simulink model "robust_tracking_nicolas"  (R2020b)
settings: Solver=VariableStepAuto  StartTime=0.0  StopTime=40.0  RelTol=1e-3
values from neighbouring files (symbols this model uses):
  drv =     [balrob_params.mat]
  g = 9.81    [balrob_params.mat]    (also in sfun_balrob_long_dyn.m)
  gbox =     [balrob_params.mat]    (also in sfun_balrob_long_dyn.m = block.DialogPrm(4).Data)
  ms22g = 0.101936799185    [balrob_params.mat]
  sens =     [balrob_params.mat]
  Ts = 0.01    [balrob_params.mat]
  wheel =     [balrob_params.mat]    (also in sfun_balrob_long_dyn.m = block.DialogPrm(5).Data)
undefined symbols (not defined in the file or in its folder): C12qq_coeff, C_gain, denHw, denLPFz, DiscIntNeverNeededParam, Fv1, g2_coeff, Ki, M11q, M12q_coeff, M22q, N_u, N_x, numHw, numLPFz, step_disturbance, step_size, T, ua2tau1
settings Model: Creator=39345  LastModifiedBy=39345
settings DataIOCC: ReturnWorkspaceOutputs=off

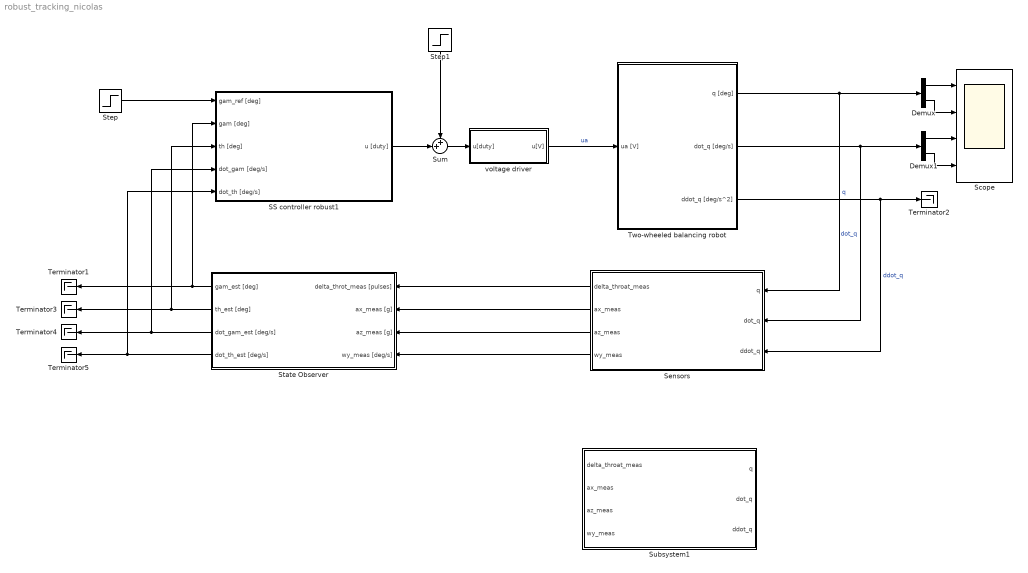
== system robust_tracking_nicolas ==
  Demux : Demux  Outputs=2
  Demux1 : Demux  Outputs=2
  SS controller robust1 : Subsystem
  Scope : Scope  NumInputPorts=4
  Sensors : Subsystem
  State Observer : Subsystem
  Step : Step  After=step_size  SampleTime=0.01
  Step1 : Step  Time=11  After=step_disturbance  SampleTime=0.01
  Subsystem1 : Subsystem
  Sum : Sum  Inputs=++|
  Terminator{1..5} (5 alike) : Terminator
  Two-wheeled balancing robot : Subsystem
  voltage driver : Subsystem
  wires:
  SS controller robust1/1(u [duty]) -> Sum/2
  State Observer/1(gam_est [deg]) -> SS controller robust1/2(gam [deg]), Terminator1/1
  State Observer/2(th_est [deg]) -> SS controller robust1/3(th [deg]), Terminator3/1
  State Observer/3(dot_gam_est [deg/s]) -> SS controller robust1/4(dot_gam [deg/s]), Terminator4/1
  State Observer/4(dot_th_est [deg/s]) -> SS controller robust1/5(dot_th [deg/s]), Terminator5/1
  Sum/1 -> voltage driver/1(u[duty])
  Demux1/1 -> Scope/3
  Sensors/1(delta_throat_meas) -> State Observer/1("delta_throt_meas [pulses] ")
  Sensors/4(wy_meas) -> State Observer/4(wy_meas [deg/s])
  Two-wheeled balancing robot/3(ddot_q [deg/s^2]) -> Sensors/3(ddot_q), Terminator2/1  "ddot_q"
  voltage driver/1(u[V]) -> Two-wheeled balancing robot/1(ua [V])  "ua"
  Demux/2 -> Scope/2
  Sensors/3(az_meas) -> State Observer/3("az_meas [g] ")
  Two-wheeled balancing robot/2(dot_q [deg/s]) -> Sensors/2(dot_q), Demux1/1  "dot_q"
  Demux1/2 -> Scope/4
  Demux/1 -> Scope/1
  Sensors/2(ax_meas) -> State Observer/2("ax_meas [g] ")
  Two-wheeled balancing robot/1(q [deg]) -> Sensors/1(q), Demux/1  "q"
  Step/1 -> SS controller robust1/1(gam_ref [deg])
  Step1/1 -> Sum/1

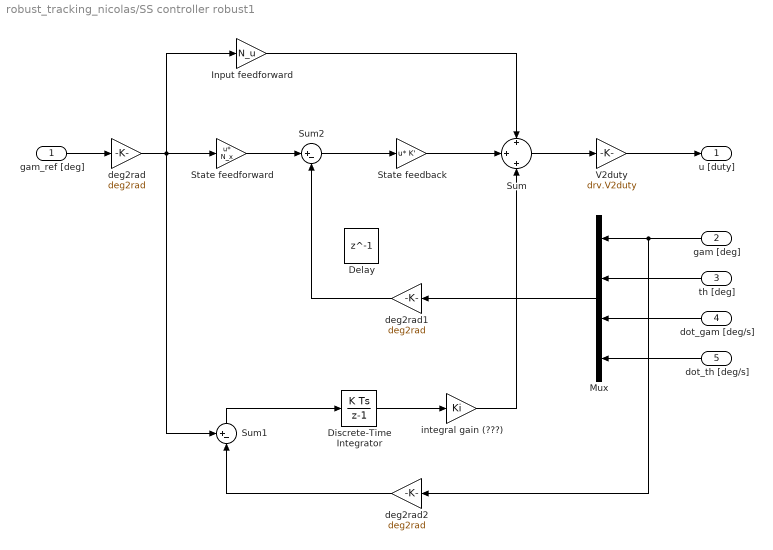
== system robust_tracking_nicolas/SS controller robust1 ==
  gam_ref [deg] : Inport
  gam [deg] : Inport  Port=2
  th [deg] : Inport  Port=3
  dot_gam [deg/s] : Inport  Port=4
  dot_th [deg/s] : Inport  Port=5
  Delay : Delay  DelayLength=1  InitialCondition=0
  Discrete-Time Integrator : DiscreteIntegrator  SampleTime=-1  ICPrevOutput=DiscIntNeverNeededParam  ICPrevScaledInput=DiscIntNeverNeededParam
  Input feedforward : Gain  Gain=N_u
  Mux : Mux
  State feedback : Gain  Gain=K'  Multiplication=Matrix(u*K)
  "State feedforward\t" : Gain  Gain=N_x  Multiplication=Matrix(u*K)
  Sum : Sum  Inputs=+|+|+
  Sum1 : Sum  Inputs=+-|
  Sum2 : Sum  Inputs=|+-
  V2duty : Gain  Gain=drv.V2duty
  deg2rad : Gain  Gain=deg2rad
  deg2rad1 : Gain  Gain=deg2rad
  deg2rad2 : Gain  Gain=deg2rad
  integral gain (???) : Gain  Gain=Ki
  u [duty] : Outport
  wires:
  gam_ref [deg]/1 -> deg2rad/1
  deg2rad/1 -> Sum1/1, "State feedforward\t"/1, Input feedforward/1
  State feedback/1 -> Sum/2
  "State feedforward\t"/1 -> Sum2/1
  Sum2/1 -> State feedback/1
  Input feedforward/1 -> Sum/1
  Sum/1 -> V2duty/1
  V2duty/1 -> u [duty]/1
  gam [deg]/1 -> deg2rad2/1, Mux/1
  Mux/1 -> deg2rad1/1
  dot_gam [deg/s]/1 -> Mux/3
  th [deg]/1 -> Mux/2
  dot_th [deg/s]/1 -> Mux/4
  deg2rad1/1 -> Sum2/2
  deg2rad2/1 -> Sum1/2
  Sum1/1 -> Discrete-Time Integrator/1
  Discrete-Time Integrator/1 -> integral gain (???)/1
  integral gain (???)/1 -> Sum/3

== system robust_tracking_nicolas/Sensors ==
  q : Inport
  dot_q : Inport  Port=2
  ddot_q : Inport  Port=3
  MPU : Subsystem
  encoder : Subsystem
  delta_throat_meas : Outport
  ax_meas : Outport  Port=2
  az_meas : Outport  Port=3
  wy_meas : Outport  Port=4
  wires:
  MPU/2(az[g]) -> az_meas/1  "az_meas"
  MPU/3(wy[deg/s]) -> wy_meas/1  "wy_meas"
  q/1 -> MPU/1(q [deg]), encoder/1(q[deg])
  ddot_q/1 -> MPU/3(ddot_q[deg/s^2])
  encoder/1(delta_throt[pulses]) -> delta_throat_meas/1  "delta_throat_meas"
  dot_q/1 -> MPU/2(dot_q [deg/s])
  MPU/1(ax[g]) -> ax_meas/1  "ax_meas"

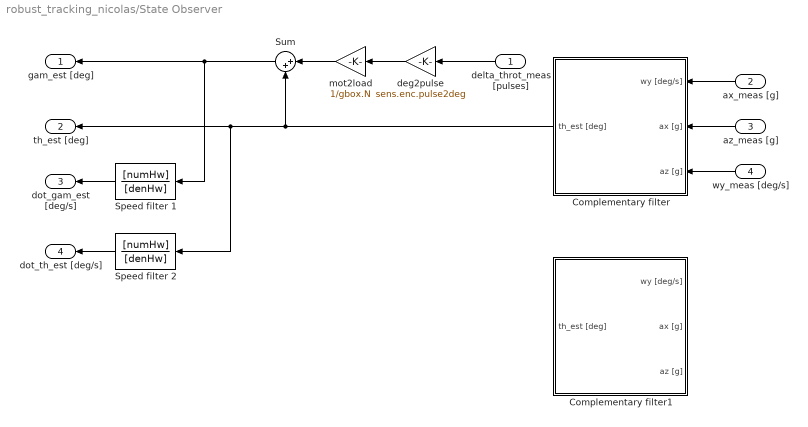
== system robust_tracking_nicolas/State Observer ==
  "delta_throt_meas [pulses] " : Inport
  "ax_meas [g] " : Inport  Port=2
  "az_meas [g] " : Inport  Port=3
  wy_meas [deg/s] : Inport  Port=4
  Complementary filter : Subsystem
  Complementary filter1 : Subsystem
  Speed filter 1 : DiscreteTransferFcn  Numerator=[numHw]  Denominator=[denHw]
  Speed filter 2 : DiscreteTransferFcn  Numerator=[numHw]  Denominator=[denHw]
  Sum : Sum  Inputs=|++
  deg2pulse : Gain  Gain=sens.enc.pulse2deg
  mot2load : Gain  Gain=1/gbox.N
  gam_est [deg] : Outport
  th_est [deg] : Outport  Port=2
  dot_gam_est [deg/s] : Outport  Port=3
  dot_th_est [deg/s] : Outport  Port=4
  wires:
  "ax_meas [g] "/1 -> Complementary filter/1(wy [deg/s])
  "az_meas [g] "/1 -> Complementary filter/2("ax [g] ")
  wy_meas [deg/s]/1 -> Complementary filter/3("az [g] ")
  deg2pulse/1 -> mot2load/1
  "delta_throt_meas [pulses] "/1 -> deg2pulse/1
  mot2load/1 -> Sum/1
  Complementary filter/1("th_est [deg] ") -> Sum/2, Speed filter 2/1, th_est [deg]/1
  Sum/1 -> Speed filter 1/1, gam_est [deg]/1
  Speed filter 1/1 -> dot_gam_est [deg/s]/1
  Speed filter 2/1 -> dot_th_est [deg/s]/1

== system robust_tracking_nicolas/Subsystem1 ==
  q : Inport
  dot_q : Inport  Port=2
  ddot_q : Inport  Port=3
  MPU : Subsystem
  encoder : Subsystem
  delta_throat_meas : Outport
  ax_meas : Outport  Port=2
  az_meas : Outport  Port=3
  wy_meas : Outport  Port=4
  wires:
  MPU/2(az[g]) -> az_meas/1  "az_meas"
  MPU/3(wy[deg/s]) -> wy_meas/1  "wy_meas"
  q/1 -> MPU/1(q [deg]), encoder/1(q[deg])
  ddot_q/1 -> MPU/3(ddot_q[deg/s^2])
  encoder/1(delta_throt[pulses]) -> delta_throat_meas/1  "delta_throat_meas"
  dot_q/1 -> MPU/2(dot_q [deg/s])
  MPU/1(ax[g]) -> ax_meas/1  "ax_meas"

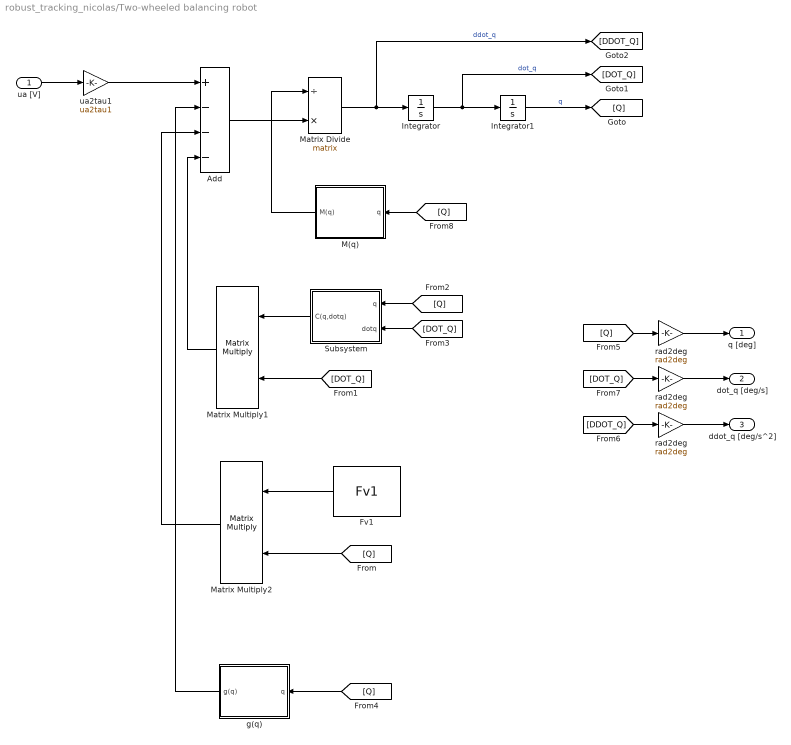
== system robust_tracking_nicolas/Two-wheeled balancing robot ==
  ua [V] : Inport
  Add : Sum  Inputs=+---
  Fv1 : Constant  Value=Fv1
  Integrator : Integrator
  Integrator1 : Integrator
  M(q) : Subsystem
  Matrix Divide : Product  Inputs=/*  Multiplication=Matrix(*)
  Matrix Multiply1 : Product  Multiplication=Matrix(*)
  Matrix Multiply2 : Product  Multiplication=Matrix(*)
  Subsystem : Subsystem
  g(q) : Subsystem
  rad2deg : Gain  Gain=rad2deg
  "rad2deg " : Gain  Gain=rad2deg
  "rad2deg  " : Gain  Gain=rad2deg
  ua2tau1 : Gain  Gain=ua2tau1
  q [deg] : Outport
  dot_q [deg/s] : Outport  Port=2
  ddot_q [deg/s^2] : Outport  Port=3
  wires:
  [DOT_Q] -> "rad2deg  "/1
  [DDOT_Q] -> "rad2deg "/1
  [Q] -> rad2deg/1
  "rad2deg  "/1 -> dot_q [deg/s]/1
  rad2deg/1 -> q [deg]/1
  "rad2deg "/1 -> ddot_q [deg/s^2]/1
  Matrix Divide/1 -> [DDOT_Q], Integrator/1  "ddot_q"
  Add/1 -> Matrix Divide/2
  [Q] -> M(q)/1(q)
  Integrator1/1 -> [Q]  "q"
  [Q] -> Subsystem/1(q)
  ua2tau1/1 -> Add/1
  Subsystem/1(C(q,dotq)) -> Matrix Multiply1/1
  [Q] -> g(q)/1(q)
  Matrix Multiply1/1 -> Add/4
  Integrator/1 -> [DOT_Q], Integrator1/1  "dot_q"
  g(q)/1(g(q)) -> Add/2
  [Q] -> Matrix Multiply2/2
  Matrix Multiply2/1 -> Add/3
  M(q)/1(M(q)) -> Matrix Divide/1
  [DOT_Q] -> Matrix Multiply1/2
  Fv1/1 -> Matrix Multiply2/1
  [DOT_Q] -> Subsystem/2(dotq)
  ua [V]/1 -> ua2tau1/1

== system robust_tracking_nicolas/voltage driver ==
  u[duty] : Inport
  Rounding Function : Rounding  Operator=fix
  Zero-Order Hold : ZeroOrderHold  SampleTime=Ts
  duty saturation : Saturate  UpperLimit=drv.dutymax  LowerLimit=-drv.dutymax
  duty2V : Gain  Gain=drv.duty2V
  voltage saturation1 : Saturate  UpperLimit=drv.Vbus  LowerLimit=-drv.Vbus
  u[V] : Outport
  wires:
  u[duty]/1 -> duty saturation/1
  duty saturation/1 -> Rounding Function/1
  Rounding Function/1 -> duty2V/1
  duty2V/1 -> voltage saturation1/1
  voltage saturation1/1 -> Zero-Order Hold/1
  Zero-Order Hold/1 -> u[V]/1

== system robust_tracking_nicolas/Sensors/MPU ==
  q [deg] : Inport
  dot_q [deg/s] : Inport  Port=2
  ddot_q[deg/s^2] : Inport  Port=3
  Accelerometer : Subsystem
  Gyroscope : Subsystem
  ax[g] : Outport
  az[g] : Outport  Port=2
  wy[deg/s] : Outport  Port=3
  wires:
  q [deg]/1 -> Accelerometer/1(q [deg])
  dot_q [deg/s]/1 -> Gyroscope/1(dot_q [deg/s]), Accelerometer/2(dot_q [deg/s])
  ddot_q[deg/s^2]/1 -> Accelerometer/3(ddot_q[deg/s^2])
  Gyroscope/1(wy[deg/s]) -> wy[deg/s]/1
  Accelerometer/1(ax[g]) -> ax[g]/1
  Accelerometer/2(az[g]) -> az[g]/1

== system robust_tracking_nicolas/Sensors/encoder ==
  q[deg] : Inport
  Demux : Demux  Outputs=2
  Subtract : Sum  Inputs=+-
  deg2pulse : Gain  Gain=sens.enc.deg2pulse
  encoder quantization : Quantizer  QuantizationInterval=sens.enc.pulse2deg
  encoder sampling : ZeroOrderHold  SampleTime=Ts
  load2mot : Gain  Gain=gbox.N
  delta_throt[pulses] : Outport
  wires:
  q[deg]/1 -> Demux/1
  Demux/1 -> Subtract/1  "gam"
  Demux/2 -> Subtract/2  "th"
  Subtract/1 -> load2mot/1
  load2mot/1 -> encoder sampling/1  "delta_throt"
  encoder sampling/1 -> encoder quantization/1
  encoder quantization/1 -> deg2pulse/1
  deg2pulse/1 -> delta_throt[pulses]/1

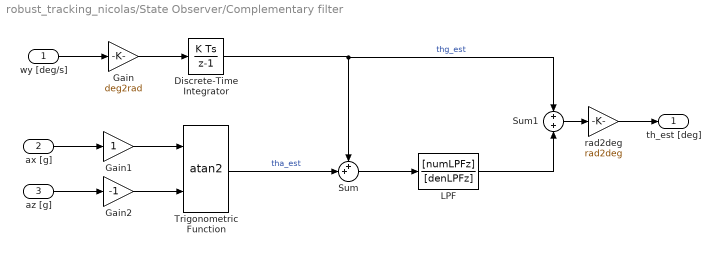
== system robust_tracking_nicolas/State Observer/Complementary filter ==
  wy [deg/s] : Inport
  "ax [g] " : Inport  Port=2
  "az [g] " : Inport  Port=3
  Discrete-Time Integrator : DiscreteIntegrator  gainval=1  SampleTime=Ts  ICPrevOutput=DiscIntNeverNeededParam  ICPrevScaledInput=DiscIntNeverNeededParam
  Gain : Gain  Gain=deg2rad
  Gain1 : Gain
  Gain2 : Gain  Gain=-1
  LPF : DiscreteTransferFcn  Numerator=[numLPFz]  Denominator=[denLPFz]
  Sum : Sum  Inputs=++|
  Sum1 : Sum
  Trigonometric Function : Trigonometry  Operator=atan2
  rad2deg : Gain  Gain=rad2deg
  "th_est [deg] " : Outport
  wires:
  "az [g] "/1 -> Gain2/1
  "ax [g] "/1 -> Gain1/1
  wy [deg/s]/1 -> Gain/1
  Gain/1 -> Discrete-Time Integrator/1
  Gain2/1 -> Trigonometric Function/2
  Gain1/1 -> Trigonometric Function/1
  Trigonometric Function/1 -> Sum/2  "tha_est"
  Discrete-Time Integrator/1 -> Sum1/1, Sum/1  "thg_est"
  rad2deg/1 -> "th_est [deg] "/1
  Sum1/1 -> rad2deg/1
  Sum/1 -> LPF/1
  LPF/1 -> Sum1/2

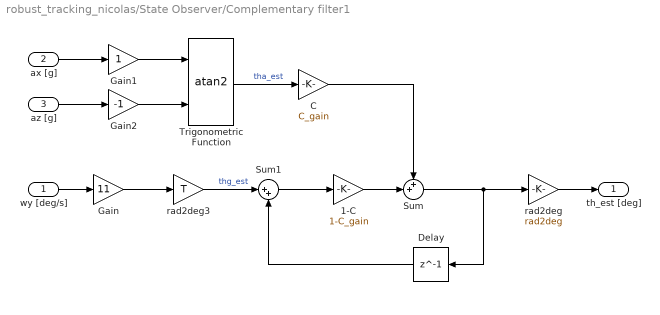
== system robust_tracking_nicolas/State Observer/Complementary filter1 ==
  wy [deg/s] : Inport
  "ax [g] " : Inport  Port=2
  "az [g] " : Inport  Port=3
  1-C : Gain  Gain=1-C_gain
  C : Gain  Gain=C_gain
  Delay : Delay  DelayLength=1
  Gain : Gain  Gain=11
  Gain1 : Gain
  Gain2 : Gain  Gain=-1
  Sum : Sum  Inputs=++|
  Sum1 : Sum  Inputs=|++
  Trigonometric Function : Trigonometry  Operator=atan2
  rad2deg : Gain  Gain=rad2deg
  rad2deg3 : Gain  Gain=T
  "th_est [deg] " : Outport
  wires:
  "az [g] "/1 -> Gain2/1
  "ax [g] "/1 -> Gain1/1
  wy [deg/s]/1 -> Gain/1
  Gain/1 -> rad2deg3/1
  Gain2/1 -> Trigonometric Function/2
  Gain1/1 -> Trigonometric Function/1
  rad2deg/1 -> "th_est [deg] "/1
  Trigonometric Function/1 -> C/1  "tha_est"
  C/1 -> Sum/1
  1-C/1 -> Sum/2
  Sum/1 -> Delay/1, rad2deg/1
  Delay/1 -> Sum1/2
  rad2deg3/1 -> Sum1/1  "thg_est"
  Sum1/1 -> 1-C/1

== system robust_tracking_nicolas/Subsystem1/MPU ==
  q [deg] : Inport
  dot_q [deg/s] : Inport  Port=2
  ddot_q[deg/s^2] : Inport  Port=3
  Accelerometer : Subsystem
  Gyroscope : Subsystem
  ax[g] : Outport
  az[g] : Outport  Port=2
  wy[deg/s] : Outport  Port=3
  wires:
  q [deg]/1 -> Accelerometer/1(q [deg])
  dot_q [deg/s]/1 -> Gyroscope/1(dot_q [deg/s]), Accelerometer/2(dot_q [deg/s])
  ddot_q[deg/s^2]/1 -> Accelerometer/3(ddot_q[deg/s^2])
  Gyroscope/1(wy[deg/s]) -> wy[deg/s]/1
  Accelerometer/1(ax[g]) -> ax[g]/1
  Accelerometer/2(az[g]) -> az[g]/1

== system robust_tracking_nicolas/Subsystem1/encoder ==
  q[deg] : Inport
  Demux : Demux  Outputs=2
  Subtract : Sum  Inputs=+-
  deg2pulse : Gain  Gain=sens.enc.deg2pulse
  encoder quantization : Quantizer  QuantizationInterval=sens.enc.pulse2deg
  encoder sampling : ZeroOrderHold  SampleTime=Ts
  load2mot : Gain  Gain=gbox.N
  delta_throt[pulses] : Outport
  wires:
  q[deg]/1 -> Demux/1
  Demux/1 -> Subtract/1  "gam"
  Demux/2 -> Subtract/2  "th"
  Subtract/1 -> load2mot/1
  load2mot/1 -> encoder sampling/1  "delta_throt"
  encoder sampling/1 -> encoder quantization/1
  encoder quantization/1 -> deg2pulse/1
  deg2pulse/1 -> delta_throt[pulses]/1

== system robust_tracking_nicolas/Two-wheeled balancing robot/M(q) ==
  q : Inport
  Constant : Constant  Value=M11q
  Constant1 : Constant  Value=M22q
  Function Caller : FunctionCaller  FunctionPrototype=y = M12q(u)  InputArgumentSpecifications=<Enter example>  OutputArgumentSpecifications=<Enter example>
  Matrix Concatenate1 : Concatenate  Mode=Multidimensional array  ConcatenateDimension=2
  Mux : Mux  Inputs=2
  Mux1 : Mux  Inputs=2
  Selector1 : Selector  InputPortWidth=2  IndexOptions=Index vector (dialog)  Indices=2  OutputSizes=1
  Simulink Function : Subsystem  TreatAsAtomicUnit=on
  M(q) : Outport
  wires:
  q/1 -> Selector1/1
  Mux1/1 -> Matrix Concatenate1/2
  Constant1/1 -> Mux1/2
  Mux/1 -> Matrix Concatenate1/1
  Function Caller/1 -> Mux/2, Mux1/1
  Matrix Concatenate1/1 -> M(q)/1
  Selector1/1 -> Function Caller/1
  Constant/1 -> Mux/1

== system robust_tracking_nicolas/Two-wheeled balancing robot/Subsystem ==
  q : Inport
  dotq : Inport  Port=2
  Constant : Constant  Value=0
  Gain : Gain  Gain=C12qq_coeff
  Matrix Concatenate1 : Concatenate  Mode=Multidimensional array  ConcatenateDimension=2
  Mux2 : Mux  Inputs=2
  Mux3 : Mux  Inputs=2
  Product : Product
  Selector1 : Selector  InputPortWidth=2  IndexOptions=Index vector (dialog)  Indices=2  OutputSizes=1
  Selector2 : Selector  InputPortWidth=2  IndexOptions=Index vector (dialog)  Indices=2  OutputSizes=1
  Trigonometric Function : Trigonometry
  C(q,dotq) : Outport
  wires:
  Mux3/1 -> Matrix Concatenate1/2
  Mux2/1 -> Matrix Concatenate1/1
  Constant/1 -> Mux3/2, Mux2/2, Mux2/1
  Matrix Concatenate1/1 -> C(q,dotq)/1
  Gain/1 -> Mux3/1
  q/1 -> Selector2/1
  dotq/1 -> Selector1/1
  Selector1/1 -> Product/2
  Product/1 -> Gain/1
  Trigonometric Function/1 -> Product/1
  Selector2/1 -> Trigonometric Function/1

== system robust_tracking_nicolas/Two-wheeled balancing robot/g(q) ==
  q : Inport
  Constant : Constant  Value=0
  Function Caller : FunctionCaller  FunctionPrototype=y = g2(u)  InputArgumentSpecifications=<Enter example>  OutputArgumentSpecifications=<Enter example>
  Mux : Mux  Inputs=2
  Selector1 : Selector  InputPortWidth=2  IndexOptions=Index vector (dialog)  Indices=2  OutputSizes=1
  Simulink Function : Subsystem  TreatAsAtomicUnit=on
  g(q) : Outport
  wires:
  q/1 -> Selector1/1
  Selector1/1 -> Function Caller/1
  Constant/1 -> Mux/1
  Function Caller/1 -> Mux/2
  Mux/1 -> g(q)/1

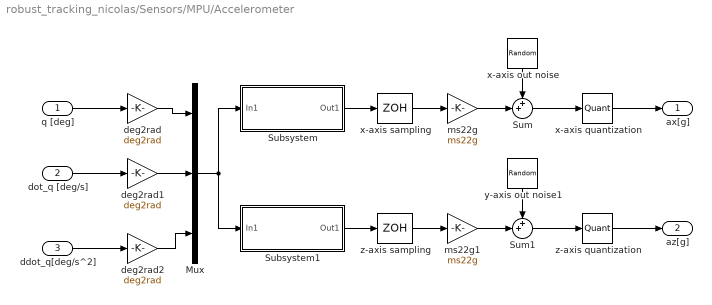
== system robust_tracking_nicolas/Sensors/MPU/Accelerometer ==
  q [deg] : Inport
  dot_q [deg/s] : Inport  Port=2
  ddot_q[deg/s^2] : Inport  Port=3
  Mux : Mux  Inputs=3
  Subsystem : Subsystem
  Subsystem1 : Subsystem
  Sum : Sum  Inputs=++|
  Sum1 : Sum  Inputs=++|
  deg2rad : Gain  Gain=deg2rad
  deg2rad1 : Gain  Gain=deg2rad
  deg2rad2 : Gain  Gain=deg2rad
  ms22g : Gain  Gain=ms22g
  ms22g1 : Gain  Gain=ms22g
  x-axis out noise : RandomNumber  Variance=sens.mpu.acc.noisevar  SampleTime=Ts
  x-axis quantization : Quantizer  QuantizationInterval=sens.mpu.acc.LSB2g
  x-axis sampling : ZeroOrderHold  SampleTime=Ts
  y-axis out noise1 : RandomNumber  Variance=sens.mpu.acc.noisevar  SampleTime=Ts
  z-axis quantization : Quantizer  QuantizationInterval=sens.mpu.acc.LSB2g
  z-axis sampling : ZeroOrderHold  SampleTime=Ts
  ax[g] : Outport
  az[g] : Outport  Port=2
  wires:
  ddot_q[deg/s^2]/1 -> deg2rad2/1
  dot_q [deg/s]/1 -> deg2rad1/1
  q [deg]/1 -> deg2rad/1
  deg2rad2/1 -> Mux/3
  deg2rad1/1 -> Mux/2
  deg2rad/1 -> Mux/1
  x-axis sampling/1 -> ms22g/1
  z-axis sampling/1 -> ms22g1/1
  x-axis out noise/1 -> Sum/1
  ms22g/1 -> Sum/2
  y-axis out noise1/1 -> Sum1/1
  ms22g1/1 -> Sum1/2
  Sum/1 -> x-axis quantization/1
  Sum1/1 -> z-axis quantization/1
  z-axis quantization/1 -> az[g]/1
  x-axis quantization/1 -> ax[g]/1
  Mux/1 -> Subsystem1/1(In1), Subsystem/1(In1)
  Subsystem/1(Out1) -> x-axis sampling/1
  Subsystem1/1(Out1) -> z-axis sampling/1

== system robust_tracking_nicolas/Sensors/MPU/Gyroscope ==
  dot_q [deg/s] : Inport
  Random Number : RandomNumber  Variance=sens.mpu.gyro.noisevar  SampleTime=Ts
  Selector2 : Selector  InputPortWidth=2  IndexOptions=Index vector (dialog)  Indices=2  OutputSizes=1
  Sum : Sum  Inputs=++|
  y-axis quantization : Quantizer  QuantizationInterval=sens.mpu.gyro.LSB2degs
  y-axis sampling : ZeroOrderHold  SampleTime=Ts
  wy[deg/s] : Outport
  wires:
  dot_q [deg/s]/1 -> Selector2/1
  Selector2/1 -> y-axis sampling/1
  y-axis sampling/1 -> Sum/2
  Random Number/1 -> Sum/1
  Sum/1 -> y-axis quantization/1
  y-axis quantization/1 -> wy[deg/s]/1

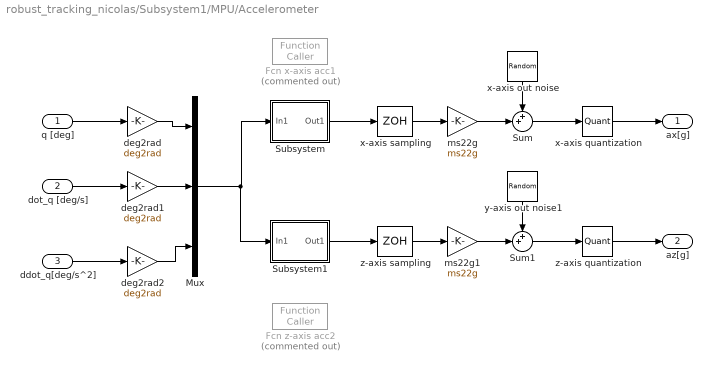
== system robust_tracking_nicolas/Subsystem1/MPU/Accelerometer ==
  q [deg] : Inport
  dot_q [deg/s] : Inport  Port=2
  ddot_q[deg/s^2] : Inport  Port=3
  Fcn x-axis acc1 : FunctionCaller  Commented=on  FunctionPrototype=y = f(u)  InputArgumentSpecifications=<Enter example>  OutputArgumentSpecifications=<Enter example>
  Fcn z-axis acc2 : FunctionCaller  Commented=on  FunctionPrototype=y = f(u)  InputArgumentSpecifications=<Enter example>  OutputArgumentSpecifications=<Enter example>
  Mux : Mux  Inputs=3
  Subsystem : Subsystem
  Subsystem1 : Subsystem
  Sum : Sum  Inputs=++|
  Sum1 : Sum  Inputs=++|
  deg2rad : Gain  Gain=deg2rad
  deg2rad1 : Gain  Gain=deg2rad
  deg2rad2 : Gain  Gain=deg2rad
  ms22g : Gain  Gain=ms22g
  ms22g1 : Gain  Gain=ms22g
  x-axis out noise : RandomNumber  Variance=sens.mpu.acc.noisevar  SampleTime=Ts
  x-axis quantization : Quantizer  QuantizationInterval=sens.mpu.acc.LSB2g
  x-axis sampling : ZeroOrderHold  SampleTime=Ts
  y-axis out noise1 : RandomNumber  Variance=sens.mpu.acc.noisevar  SampleTime=Ts
  z-axis quantization : Quantizer  QuantizationInterval=sens.mpu.acc.LSB2g
  z-axis sampling : ZeroOrderHold  SampleTime=Ts
  ax[g] : Outport
  az[g] : Outport  Port=2
  wires:
  ddot_q[deg/s^2]/1 -> deg2rad2/1
  dot_q [deg/s]/1 -> deg2rad1/1
  q [deg]/1 -> deg2rad/1
  deg2rad2/1 -> Mux/3
  deg2rad1/1 -> Mux/2
  deg2rad/1 -> Mux/1
  Mux/1 -> Subsystem1/1(In1), Subsystem/1(In1)
  Subsystem1/1(Out1) -> z-axis sampling/1
  Subsystem/1(Out1) -> x-axis sampling/1
  x-axis sampling/1 -> ms22g/1
  z-axis sampling/1 -> ms22g1/1
  x-axis out noise/1 -> Sum/1
  ms22g/1 -> Sum/2
  y-axis out noise1/1 -> Sum1/1
  ms22g1/1 -> Sum1/2
  Sum/1 -> x-axis quantization/1
  Sum1/1 -> z-axis quantization/1
  z-axis quantization/1 -> az[g]/1
  x-axis quantization/1 -> ax[g]/1

== system robust_tracking_nicolas/Subsystem1/MPU/Gyroscope ==
  dot_q [deg/s] : Inport
  Random Number : RandomNumber  Variance=sens.mpu.gyro.noisevar  SampleTime=Ts
  Selector1 : Selector  InputPortWidth=3  IndexOptions=Index vector (dialog)  Indices=[1 3]  OutputSizes=1
  Sum : Sum  Inputs=++|
  y-axis quantization : Quantizer  QuantizationInterval=sens.mpu.gyro.LSB2degs
  y-axis sampling : ZeroOrderHold  SampleTime=Ts
  wy[deg/s] : Outport
  wires:
  dot_q [deg/s]/1 -> Selector1/1
  Selector1/1 -> y-axis sampling/1
  y-axis sampling/1 -> Sum/2
  Random Number/1 -> Sum/1
  Sum/1 -> y-axis quantization/1
  y-axis quantization/1 -> wy[deg/s]/1

== system robust_tracking_nicolas/Two-wheeled balancing robot/M(q)/Simulink Function ==
  f : TriggerPort  TriggerType=function-call  IsSimulinkFunction=on  FunctionName=M12q  FunctionVisibility=scoped  VariantControl=(inherit)
  Gain : Gain  Gain=M12q_coeff
  Trigonometric Function : Trigonometry  Operator=cos
  u : ArgIn  DisableCoverage=on  ArgumentName=u
  y : ArgOut  DisableCoverage=on  ArgumentName=y
  wires:
  u/1 -> Trigonometric Function/1
  Trigonometric Function/1 -> Gain/1
  Gain/1 -> y/1

== system robust_tracking_nicolas/Two-wheeled balancing robot/g(q)/Simulink Function ==
  f : TriggerPort  TriggerType=function-call  IsSimulinkFunction=on  FunctionName=g2  FunctionVisibility=scoped  VariantControl=(inherit)
  Gain : Gain  Gain=g2_coeff
  Trigonometric Function : Trigonometry
  u : ArgIn  DisableCoverage=on  ArgumentName=u
  y : ArgOut  DisableCoverage=on  ArgumentName=y
  wires:
  u/1 -> Trigonometric Function/1
  Trigonometric Function/1 -> Gain/1
  Gain/1 -> y/1

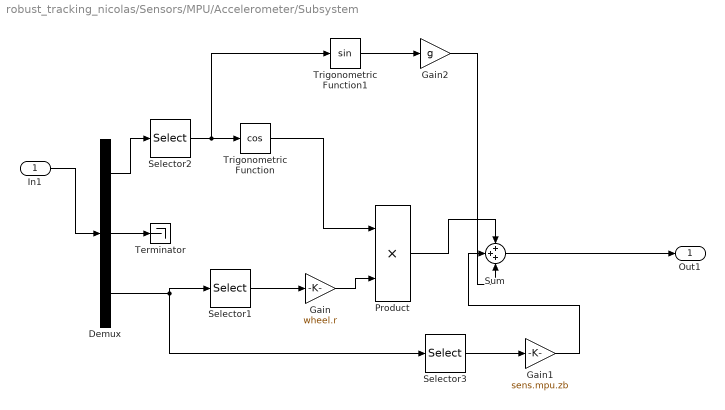
== system robust_tracking_nicolas/Sensors/MPU/Accelerometer/Subsystem ==
  In1 : Inport
  Demux : Demux  Outputs=3
  Gain : Gain  Gain=wheel.r
  Gain1 : Gain  Gain=sens.mpu.zb
  Gain2 : Gain  Gain=g
  Product : Product
  Selector1 : Selector  InputPortWidth=2  IndexOptions=Index vector (dialog)  Indices=1  OutputSizes=1
  Selector2 : Selector  InputPortWidth=2  IndexOptions=Index vector (dialog)  Indices=2  OutputSizes=1
  Selector3 : Selector  InputPortWidth=2  IndexOptions=Index vector (dialog)  Indices=2  OutputSizes=1
  Sum : Sum  Inputs=+++
  Terminator : Terminator
  Trigonometric Function : Trigonometry  Operator=cos
  Trigonometric Function1 : Trigonometry
  Out1 : Outport
  wires:
  In1/1 -> Demux/1
  Demux/3 -> Selector3/1, Selector1/1
  Selector1/1 -> Gain/1
  Demux/1 -> Selector2/1
  Selector2/1 -> Trigonometric Function1/1, Trigonometric Function/1
  Gain/1 -> Product/2
  Trigonometric Function/1 -> Product/1
  Product/1 -> Sum/1
  Sum/1 -> Out1/1
  Selector3/1 -> Gain1/1
  Trigonometric Function1/1 -> Gain2/1
  Gain1/1 -> Sum/2
  Gain2/1 -> Sum/3
  Demux/2 -> Terminator/1

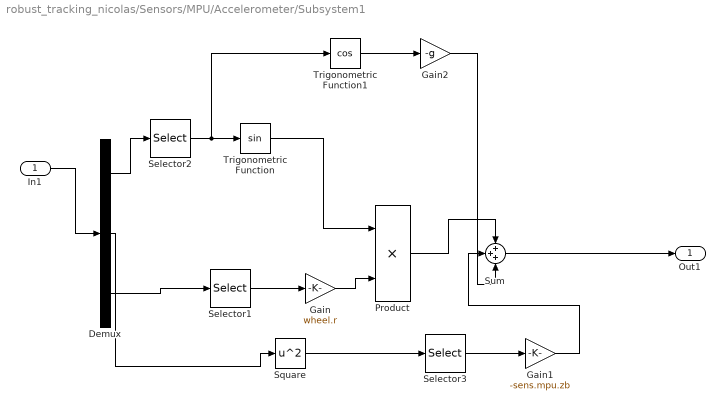
== system robust_tracking_nicolas/Sensors/MPU/Accelerometer/Subsystem1 ==
  In1 : Inport
  Demux : Demux  Outputs=3
  Gain : Gain  Gain=wheel.r
  Gain1 : Gain  Gain=-sens.mpu.zb
  Gain2 : Gain  Gain=-g
  Product : Product
  Selector1 : Selector  InputPortWidth=2  IndexOptions=Index vector (dialog)  Indices=1  OutputSizes=1
  Selector2 : Selector  InputPortWidth=2  IndexOptions=Index vector (dialog)  Indices=2  OutputSizes=1
  Selector3 : Selector  InputPortWidth=2  IndexOptions=Index vector (dialog)  Indices=2  OutputSizes=1
  Square : Math  Operator=square  SaturateOnIntegerOverflow=on
  Sum : Sum  Inputs=+++
  Trigonometric Function : Trigonometry
  Trigonometric Function1 : Trigonometry  Operator=cos
  Out1 : Outport
  wires:
  Selector1/1 -> Gain/1
  In1/1 -> Demux/1
  Demux/1 -> Selector2/1
  Selector3/1 -> Gain1/1
  Gain2/1 -> Sum/3
  Gain/1 -> Product/2
  Gain1/1 -> Sum/2
  Selector2/1 -> Trigonometric Function1/1, Trigonometric Function/1
  Trigonometric Function1/1 -> Gain2/1
  Trigonometric Function/1 -> Product/1
  Sum/1 -> Out1/1
  Product/1 -> Sum/1
  Demux/3 -> Selector1/1
  Demux/2 -> Square/1
  Square/1 -> Selector3/1

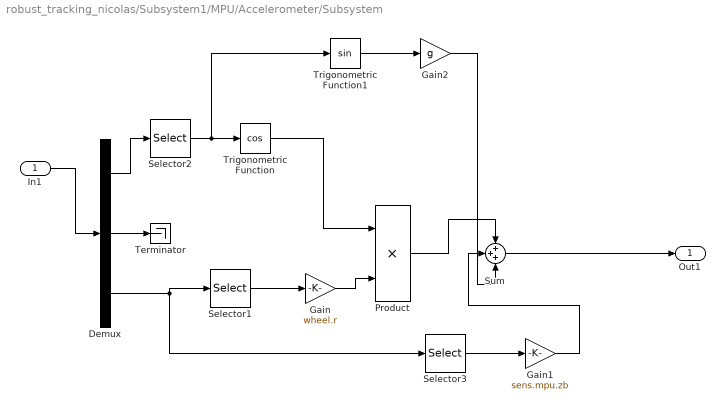
== system robust_tracking_nicolas/Subsystem1/MPU/Accelerometer/Subsystem ==
  In1 : Inport
  Demux : Demux  Outputs=3
  Gain : Gain  Gain=wheel.r
  Gain1 : Gain  Gain=sens.mpu.zb
  Gain2 : Gain  Gain=g
  Product : Product
  Selector1 : Selector  InputPortWidth=2  IndexOptions=Index vector (dialog)  Indices=1  OutputSizes=1
  Selector2 : Selector  InputPortWidth=2  IndexOptions=Index vector (dialog)  Indices=2  OutputSizes=1
  Selector3 : Selector  InputPortWidth=2  IndexOptions=Index vector (dialog)  Indices=2  OutputSizes=1
  Sum : Sum  Inputs=+++
  Terminator : Terminator
  Trigonometric Function : Trigonometry  Operator=cos
  Trigonometric Function1 : Trigonometry
  Out1 : Outport
  wires:
  In1/1 -> Demux/1
  Demux/3 -> Selector3/1, Selector1/1
  Selector1/1 -> Gain/1
  Demux/1 -> Selector2/1
  Selector2/1 -> Trigonometric Function1/1, Trigonometric Function/1
  Gain/1 -> Product/2
  Trigonometric Function/1 -> Product/1
  Product/1 -> Sum/1
  Sum/1 -> Out1/1
  Selector3/1 -> Gain1/1
  Trigonometric Function1/1 -> Gain2/1
  Gain1/1 -> Sum/2
  Gain2/1 -> Sum/3
  Demux/2 -> Terminator/1

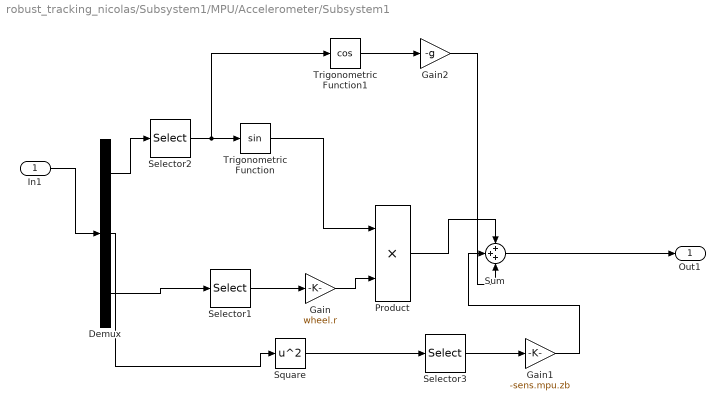
== system robust_tracking_nicolas/Subsystem1/MPU/Accelerometer/Subsystem1 ==
  In1 : Inport
  Demux : Demux  Outputs=3
  Gain : Gain  Gain=wheel.r
  Gain1 : Gain  Gain=-sens.mpu.zb
  Gain2 : Gain  Gain=-g
  Product : Product
  Selector1 : Selector  InputPortWidth=2  IndexOptions=Index vector (dialog)  Indices=1  OutputSizes=1
  Selector2 : Selector  InputPortWidth=2  IndexOptions=Index vector (dialog)  Indices=2  OutputSizes=1
  Selector3 : Selector  InputPortWidth=2  IndexOptions=Index vector (dialog)  Indices=2  OutputSizes=1
  Square : Math  Operator=square  SaturateOnIntegerOverflow=on
  Sum : Sum  Inputs=+++
  Trigonometric Function : Trigonometry
  Trigonometric Function1 : Trigonometry  Operator=cos
  Out1 : Outport
  wires:
  Selector1/1 -> Gain/1
  In1/1 -> Demux/1
  Demux/1 -> Selector2/1
  Selector3/1 -> Gain1/1
  Gain2/1 -> Sum/3
  Gain/1 -> Product/2
  Gain1/1 -> Sum/2
  Selector2/1 -> Trigonometric Function1/1, Trigonometric Function/1
  Trigonometric Function1/1 -> Gain2/1
  Trigonometric Function/1 -> Product/1
  Sum/1 -> Out1/1
  Product/1 -> Sum/1
  Demux/3 -> Selector1/1
  Demux/2 -> Square/1
  Square/1 -> Selector3/1
